simulink model "segmentCalc"  (R2019a)
settings: Solver=VariableStepAuto  StartTime=0.0  StopTime=5  FixedStep=1  RelTol=1e-3
undefined symbols (not defined in the file or in its folder): ggV, init, segments
settings Model: Creator=Frieder Uerlings  LastModifiedBy=Frieder Uerlings

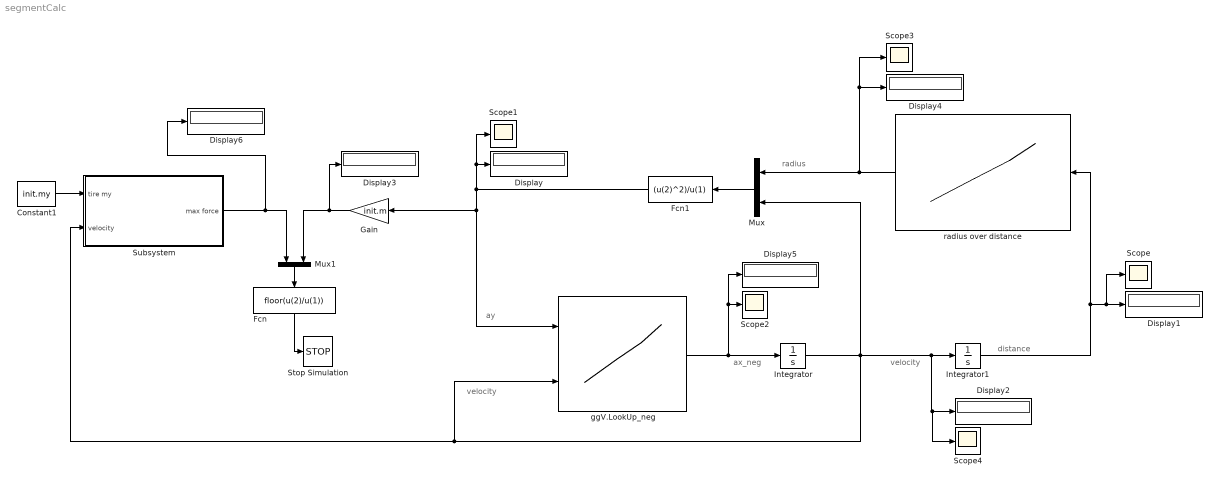
== system segmentCalc ==
  note: radius
  note: distance
  note: velocity
  note: velocity
  note: ay
  note: ax_neg
  Constant1 : Constant  Value=init.my
  Display{,1..6} (7 alike) : Display
  Fcn : Fcn  Expr=floor(u(2)/u(1))
  Fcn1 : Fcn  Expr=(u(2)^2)/u(1)
  Gain : Gain  Gain=init.m
  Integrator : Integrator  InitialCondition=16.2386865113317
  Integrator1 : Integrator
  Mux : Mux  Inputs=2
  Mux1 : Mux  Inputs=2
  Scope{,1..4} (5 alike) : Scope
  Stop Simulation : Stop
  Subsystem : Subsystem
  ggV.LookUp_neg : Lookup_n-D  BreakpointsForDimension1=[1:1:ggV.interpMax+1]  BreakpointsForDimension2=[0:init.deltaV:init.maxV]  Table=ggV.LookUp_pos(:,:)  InternalRulePriority=Speed  RndMeth=Simplest  InputSameDT=on
  radius over distance : Lookup_n-D  NumberOfTableDimensions=1  BreakpointsForDimension1=[0:1:38]  Table=segments{1,1}  InternalRulePriority=Speed  RndMeth=Simplest  InputSameDT=on
  wires:
  Integrator1/1 -> Scope/1, Display1/1, radius over distance/1
  ggV.LookUp_neg/1 -> Scope2/1, Display5/1, Integrator/1
  Integrator/1 -> Mux/2, Scope4/1, Display2/1, Integrator1/1, ggV.LookUp_neg/2, Subsystem/2(velocity)
  radius over distance/1 -> Scope3/1, Display4/1, Mux/1
  Mux/1 -> Fcn1/1
  Fcn1/1 -> Gain/1, ggV.LookUp_neg/1, Display/1, Scope1/1
  Constant1/1 -> Subsystem/1(tire my)
  Subsystem/1(max force) -> Display6/1, Mux1/1
  Gain/1 -> Display3/1, Mux1/2
  Mux1/1 -> Fcn/1
  Fcn/1 -> Stop Simulation/1

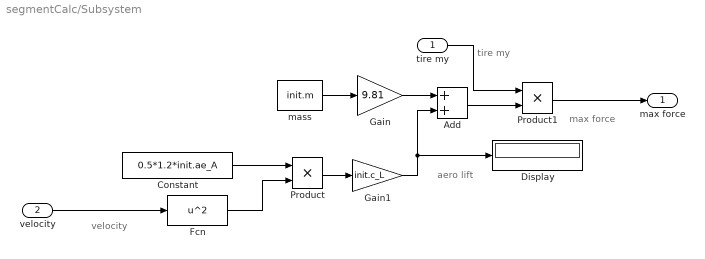
== system segmentCalc/Subsystem ==
  note: max force
  note: aero lift
  note: tire my
  note: velocity
  tire my : Inport
  velocity : Inport  Port=2
  Add : Sum
  Constant : Constant  Value=0.5*1.2*init.ae_A
  Display : Display
  Fcn : Fcn  Expr=u^2
  Gain : Gain  Gain=9.81
  Gain1 : Gain  Gain=init.c_L
  Product : Product
  Product1 : Product
  "mass " : Constant  Value=init.m
  max force : Outport
  wires:
  Constant/1 -> Product/1
  Add/1 -> Product1/2
  "mass "/1 -> Gain/1
  Fcn/1 -> Product/2
  Product1/1 -> max force/1
  Gain/1 -> Add/1
  Product/1 -> Gain1/1
  tire my/1 -> Product1/1
  velocity/1 -> Fcn/1
  Gain1/1 -> Add/2, Display/1
